simulink library "INT_EISGov_SelectParameter"  (R2016b)
settings: Solver=VariableStepAuto  StartTime=0.0  StopTime=10.0  RelTol=1e-3
settings Model: Creator=xuxingpei  LastModifiedBy=xuxingpei

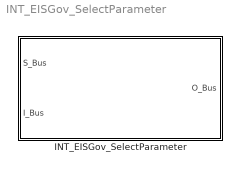
== system INT_EISGov_SelectParameter ==
  INT_EISGov_SelectParameter : Subsystem

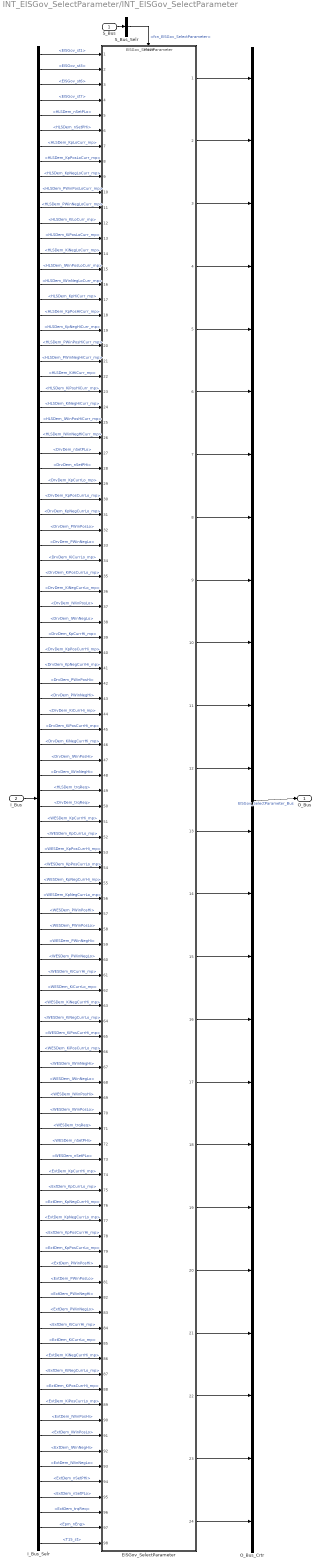
== system INT_EISGov_SelectParameter/INT_EISGov_SelectParameter ==
  S_Bus : Inport
  I_Bus : Inport  Port=2
  EISGov_SelectParameter : ModelReference  ModelNameDialog=EISGov_SelectParameter  SimulationMode=Normal  ModelReferenceVersion=1.180  TriggerPortName=function  TriggerPortTriggerType=function-call  TriggerPortStatesWhenEnabling=held
  I_Bus_Selr : BusSelector  OutputSignals=EISGov_st1,EISGov_st3,EISGov_st6,EISGov_st7,HLSDem_nSetPLo,HLSDem_nSetPHi,HLSDem_KpLoCurr_mp,HLSDem_KpPosLoCurr_mp,HLSDem_KpNegLoCurr_mp,HLSDem_PWinPosLoCurr_mp,HLSDem_PWinNegLoCurr_mp,HLSDem_KiLoCurr_mp,HLSDem_KiPosLoCurr_mp,HLSDem_KiNegLoCurr_mp,HLSDem_IWinPosLoCurr_mp,HLSDem_IWinNegLoCurr_mp,HLSDem_KpHiCurr_mp,HLSDem_KpPosHiCurr_mp,HLSDem_KpNegHiCurr_mp,HLSDem_PWinPosHiCurr_mp,HLSDem_PWinNegHiCurr_mp,HLSDem_KiHiCurr_mp,HLSDem_KiPosHiCurr_mp,HLSDem_KiNegHiCurr_mp,HLSDem_IWinPosHiCurr_mp,HLSDem_IWinNegHiCurr_mp,DrvDem_nSetPLo,DrvDem_nSetPHi,DrvDem_KpCurrLo_mp,DrvDem_KpPosCurrLo_mp,DrvDem_KpNegCurrLo_mp,DrvDem_PWinPosLo,DrvDem_PWinNegLo,DrvDem_KiCurrLo_mp,DrvDem_KiPosCurrLo_mp,DrvDem_KiNegCurrLo_mp,DrvDem_IWinPosLo,DrvDem_IWinNegLo,DrvDem_KpCurrHi_mp,DrvDem_KpPosCurrHi_mp,DrvDem_KpNegCurrHi_mp,DrvDem_PWinPosHi,DrvDem_PWinNegHi,DrvDem_KiCurrHi_mp,DrvDem_KiPosCurrHi_mp,DrvDem_KiNegCurrHi_mp,DrvDem_IWinPosHi,DrvDem_IWinNegHi,HLSDem_trqReq,DrvDem_trqReq,WESDem_KpCurrHi_mp,WESDem_KpCurrLo_mp,WESDem_KpPosCurrHi_mp,WESDem_KpPosCurrLo_mp,WESDem_KpNegCurrHi_mp,WESDem_KpNegCurrLo_mp,WESDem_PWinPosHi,WESDem_PWinPosLo,WESDem_PWinNegHi,WESDem_PWinNegLo,WESDem_KiCurrHi_mp,WESDem_KiCurrLo_mp,WESDem_KiNegCurrHi_mp,WESDem_KiNegCurrLo_mp,WESDem_KiPosCurrHi_mp,WESDem_KiPosCurrLo_mp,WESDem_IWinNegHi,WESDem_IWinNegLo,WESDem_IWinPosHi,WESDem_IWinPosLo,WESDem_trqReq,WESDem_nSetPHi,WESDem_nSetPLo,ExtDem_KpCurrHi_mp,ExtDem_KpCurrLo_mp,ExtDem_KpNegCurrHi_mp,ExtDem_KpNegCurrLo_mp,ExtDem_KpPosCurrHi_mp,ExtDem_KpPosCurrLo_mp,ExtDem_PWinPosHi,ExtDem_PWinPosLo,ExtDem_PWinNegHi,ExtDem_PWinNegLo,ExtDem_KiCurrHi_mp,ExtDem_KiCurrLo_mp,ExtDem_KiNegCurrHi_mp,ExtDem_KiNegCurrLo_mp,ExtDem_KiPosCurrHi_mp,ExtDem_KiPosCurrLo_mp,ExtDem_IWinPosHi,ExtDem_IWinPosLo,ExtDem_IWinNegHi,ExtDem_IWinNegLo,ExtDem_nSetPHi,ExtDem_nSetPLo,ExtDem_trqReq,Epm_nEng,T15_st
  O_Bus_Crtr : BusCreator  Inputs=24
  S_Bus_Selr : BusSelector  OutputSignals=fcn_EISGov_SelectParameter
  O_Bus : Outport
  wires:
  S_Bus_Selr/1 -> EISGov_SelectParameter/Trigger  "<fcn_EISGov_SelectParameter>"
  S_Bus/1 -> S_Bus_Selr/1
  I_Bus/1 -> I_Bus_Selr/1
  I_Bus_Selr/1 -> EISGov_SelectParameter/1  "<EISGov_st1>"
  I_Bus_Selr/2 -> EISGov_SelectParameter/2  "<EISGov_st3>"
  I_Bus_Selr/3 -> EISGov_SelectParameter/3  "<EISGov_st6>"
  I_Bus_Selr/4 -> EISGov_SelectParameter/4  "<EISGov_st7>"
  I_Bus_Selr/5 -> EISGov_SelectParameter/5  "<HLSDem_nSetPLo>"
  I_Bus_Selr/6 -> EISGov_SelectParameter/6  "<HLSDem_nSetPHi>"
  I_Bus_Selr/7 -> EISGov_SelectParameter/7  "<HLSDem_KpLoCurr_mp>"
  I_Bus_Selr/8 -> EISGov_SelectParameter/8  "<HLSDem_KpPosLoCurr_mp>"
  I_Bus_Selr/9 -> EISGov_SelectParameter/9  "<HLSDem_KpNegLoCurr_mp>"
  I_Bus_Selr/10 -> EISGov_SelectParameter/10  "<HLSDem_PWinPosLoCurr_mp>"
  I_Bus_Selr/11 -> EISGov_SelectParameter/11  "<HLSDem_PWinNegLoCurr_mp>"
  I_Bus_Selr/12 -> EISGov_SelectParameter/12  "<HLSDem_KiLoCurr_mp>"
  I_Bus_Selr/13 -> EISGov_SelectParameter/13  "<HLSDem_KiPosLoCurr_mp>"
  I_Bus_Selr/14 -> EISGov_SelectParameter/14  "<HLSDem_KiNegLoCurr_mp>"
  I_Bus_Selr/15 -> EISGov_SelectParameter/15  "<HLSDem_IWinPosLoCurr_mp>"
  I_Bus_Selr/16 -> EISGov_SelectParameter/16  "<HLSDem_IWinNegLoCurr_mp>"
  I_Bus_Selr/17 -> EISGov_SelectParameter/17  "<HLSDem_KpHiCurr_mp>"
  I_Bus_Selr/18 -> EISGov_SelectParameter/18  "<HLSDem_KpPosHiCurr_mp>"
  I_Bus_Selr/19 -> EISGov_SelectParameter/19  "<HLSDem_KpNegHiCurr_mp>"
  I_Bus_Selr/20 -> EISGov_SelectParameter/20  "<HLSDem_PWinPosHiCurr_mp>"
  I_Bus_Selr/21 -> EISGov_SelectParameter/21  "<HLSDem_PWinNegHiCurr_mp>"
  I_Bus_Selr/22 -> EISGov_SelectParameter/22  "<HLSDem_KiHiCurr_mp>"
  I_Bus_Selr/23 -> EISGov_SelectParameter/23  "<HLSDem_KiPosHiCurr_mp>"
  I_Bus_Selr/24 -> EISGov_SelectParameter/24  "<HLSDem_KiNegHiCurr_mp>"
  I_Bus_Selr/25 -> EISGov_SelectParameter/25  "<HLSDem_IWinPosHiCurr_mp>"
  I_Bus_Selr/26 -> EISGov_SelectParameter/26  "<HLSDem_IWinNegHiCurr_mp>"
  I_Bus_Selr/27 -> EISGov_SelectParameter/27  "<DrvDem_nSetPLo>"
  I_Bus_Selr/28 -> EISGov_SelectParameter/28  "<DrvDem_nSetPHi>"
  I_Bus_Selr/29 -> EISGov_SelectParameter/29  "<DrvDem_KpCurrLo_mp>"
  I_Bus_Selr/30 -> EISGov_SelectParameter/30  "<DrvDem_KpPosCurrLo_mp>"
  I_Bus_Selr/31 -> EISGov_SelectParameter/31  "<DrvDem_KpNegCurrLo_mp>"
  I_Bus_Selr/32 -> EISGov_SelectParameter/32  "<DrvDem_PWinPosLo>"
  I_Bus_Selr/33 -> EISGov_SelectParameter/33  "<DrvDem_PWinNegLo>"
  I_Bus_Selr/34 -> EISGov_SelectParameter/34  "<DrvDem_KiCurrLo_mp>"
  I_Bus_Selr/35 -> EISGov_SelectParameter/35  "<DrvDem_KiPosCurrLo_mp>"
  I_Bus_Selr/36 -> EISGov_SelectParameter/36  "<DrvDem_KiNegCurrLo_mp>"
  I_Bus_Selr/37 -> EISGov_SelectParameter/37  "<DrvDem_IWinPosLo>"
  I_Bus_Selr/38 -> EISGov_SelectParameter/38  "<DrvDem_IWinNegLo>"
  I_Bus_Selr/39 -> EISGov_SelectParameter/39  "<DrvDem_KpCurrHi_mp>"
  I_Bus_Selr/40 -> EISGov_SelectParameter/40  "<DrvDem_KpPosCurrHi_mp>"
  I_Bus_Selr/41 -> EISGov_SelectParameter/41  "<DrvDem_KpNegCurrHi_mp>"
  I_Bus_Selr/42 -> EISGov_SelectParameter/42  "<DrvDem_PWinPosHi>"
  I_Bus_Selr/43 -> EISGov_SelectParameter/43  "<DrvDem_PWinNegHi>"
  I_Bus_Selr/44 -> EISGov_SelectParameter/44  "<DrvDem_KiCurrHi_mp>"
  I_Bus_Selr/45 -> EISGov_SelectParameter/45  "<DrvDem_KiPosCurrHi_mp>"
  I_Bus_Selr/46 -> EISGov_SelectParameter/46  "<DrvDem_KiNegCurrHi_mp>"
  I_Bus_Selr/47 -> EISGov_SelectParameter/47  "<DrvDem_IWinPosHi>"
  I_Bus_Selr/48 -> EISGov_SelectParameter/48  "<DrvDem_IWinNegHi>"
  I_Bus_Selr/49 -> EISGov_SelectParameter/49  "<HLSDem_trqReq>"
  I_Bus_Selr/50 -> EISGov_SelectParameter/50  "<DrvDem_trqReq>"
  I_Bus_Selr/51 -> EISGov_SelectParameter/51  "<WESDem_KpCurrHi_mp>"
  I_Bus_Selr/52 -> EISGov_SelectParameter/52  "<WESDem_KpCurrLo_mp>"
  I_Bus_Selr/53 -> EISGov_SelectParameter/53  "<WESDem_KpPosCurrHi_mp>"
  I_Bus_Selr/54 -> EISGov_SelectParameter/54  "<WESDem_KpPosCurrLo_mp>"
  I_Bus_Selr/55 -> EISGov_SelectParameter/55  "<WESDem_KpNegCurrHi_mp>"
  I_Bus_Selr/56 -> EISGov_SelectParameter/56  "<WESDem_KpNegCurrLo_mp>"
  I_Bus_Selr/57 -> EISGov_SelectParameter/57  "<WESDem_PWinPosHi>"
  I_Bus_Selr/58 -> EISGov_SelectParameter/58  "<WESDem_PWinPosLo>"
  I_Bus_Selr/59 -> EISGov_SelectParameter/59  "<WESDem_PWinNegHi>"
  I_Bus_Selr/60 -> EISGov_SelectParameter/60  "<WESDem_PWinNegLo>"
  I_Bus_Selr/61 -> EISGov_SelectParameter/61  "<WESDem_KiCurrHi_mp>"
  I_Bus_Selr/62 -> EISGov_SelectParameter/62  "<WESDem_KiCurrLo_mp>"
  I_Bus_Selr/63 -> EISGov_SelectParameter/63  "<WESDem_KiNegCurrHi_mp>"
  I_Bus_Selr/64 -> EISGov_SelectParameter/64  "<WESDem_KiNegCurrLo_mp>"
  I_Bus_Selr/65 -> EISGov_SelectParameter/65  "<WESDem_KiPosCurrHi_mp>"
  I_Bus_Selr/66 -> EISGov_SelectParameter/66  "<WESDem_KiPosCurrLo_mp>"
  I_Bus_Selr/67 -> EISGov_SelectParameter/67  "<WESDem_IWinNegHi>"
  I_Bus_Selr/68 -> EISGov_SelectParameter/68  "<WESDem_IWinNegLo>"
  I_Bus_Selr/69 -> EISGov_SelectParameter/69  "<WESDem_IWinPosHi>"
  I_Bus_Selr/70 -> EISGov_SelectParameter/70  "<WESDem_IWinPosLo>"
  I_Bus_Selr/71 -> EISGov_SelectParameter/71  "<WESDem_trqReq>"
  I_Bus_Selr/72 -> EISGov_SelectParameter/72  "<WESDem_nSetPHi>"
  I_Bus_Selr/73 -> EISGov_SelectParameter/73  "<WESDem_nSetPLo>"
  I_Bus_Selr/74 -> EISGov_SelectParameter/74  "<ExtDem_KpCurrHi_mp>"
  I_Bus_Selr/75 -> EISGov_SelectParameter/75  "<ExtDem_KpCurrLo_mp>"
  I_Bus_Selr/76 -> EISGov_SelectParameter/76  "<ExtDem_KpNegCurrHi_mp>"
  I_Bus_Selr/77 -> EISGov_SelectParameter/77  "<ExtDem_KpNegCurrLo_mp>"
  I_Bus_Selr/78 -> EISGov_SelectParameter/78  "<ExtDem_KpPosCurrHi_mp>"
  I_Bus_Selr/79 -> EISGov_SelectParameter/79  "<ExtDem_KpPosCurrLo_mp>"
  I_Bus_Selr/80 -> EISGov_SelectParameter/80  "<ExtDem_PWinPosHi>"
  I_Bus_Selr/81 -> EISGov_SelectParameter/81  "<ExtDem_PWinPosLo>"
  I_Bus_Selr/82 -> EISGov_SelectParameter/82  "<ExtDem_PWinNegHi>"
  I_Bus_Selr/83 -> EISGov_SelectParameter/83  "<ExtDem_PWinNegLo>"
  I_Bus_Selr/84 -> EISGov_SelectParameter/84  "<ExtDem_KiCurrHi_mp>"
  I_Bus_Selr/85 -> EISGov_SelectParameter/85  "<ExtDem_KiCurrLo_mp>"
  I_Bus_Selr/86 -> EISGov_SelectParameter/86  "<ExtDem_KiNegCurrHi_mp>"
  I_Bus_Selr/87 -> EISGov_SelectParameter/87  "<ExtDem_KiNegCurrLo_mp>"
  I_Bus_Selr/88 -> EISGov_SelectParameter/88  "<ExtDem_KiPosCurrHi_mp>"
  I_Bus_Selr/89 -> EISGov_SelectParameter/89  "<ExtDem_KiPosCurrLo_mp>"
  I_Bus_Selr/90 -> EISGov_SelectParameter/90  "<ExtDem_IWinPosHi>"
  I_Bus_Selr/91 -> EISGov_SelectParameter/91  "<ExtDem_IWinPosLo>"
  I_Bus_Selr/92 -> EISGov_SelectParameter/92  "<ExtDem_IWinNegHi>"
  I_Bus_Selr/93 -> EISGov_SelectParameter/93  "<ExtDem_IWinNegLo>"
  I_Bus_Selr/94 -> EISGov_SelectParameter/94  "<ExtDem_nSetPHi>"
  I_Bus_Selr/95 -> EISGov_SelectParameter/95  "<ExtDem_nSetPLo>"
  I_Bus_Selr/96 -> EISGov_SelectParameter/96  "<ExtDem_trqReq>"
  I_Bus_Selr/97 -> EISGov_SelectParameter/97  "<Epm_nEng>"
  I_Bus_Selr/98 -> EISGov_SelectParameter/98  "<T15_st>"
  O_Bus_Crtr/1 -> O_Bus/1  "EISGov_SelectParameter_Bus"
  EISGov_SelectParameter/1 -> O_Bus_Crtr/1
  EISGov_SelectParameter/2 -> O_Bus_Crtr/2
  EISGov_SelectParameter/3 -> O_Bus_Crtr/3
  EISGov_SelectParameter/4 -> O_Bus_Crtr/4
  EISGov_SelectParameter/5 -> O_Bus_Crtr/5
  EISGov_SelectParameter/6 -> O_Bus_Crtr/6
  EISGov_SelectParameter/7 -> O_Bus_Crtr/7
  EISGov_SelectParameter/8 -> O_Bus_Crtr/8
  EISGov_SelectParameter/9 -> O_Bus_Crtr/9
  EISGov_SelectParameter/10 -> O_Bus_Crtr/10
  EISGov_SelectParameter/11 -> O_Bus_Crtr/11
  EISGov_SelectParameter/12 -> O_Bus_Crtr/12
  EISGov_SelectParameter/13 -> O_Bus_Crtr/13
  EISGov_SelectParameter/14 -> O_Bus_Crtr/14
  EISGov_SelectParameter/15 -> O_Bus_Crtr/15
  EISGov_SelectParameter/16 -> O_Bus_Crtr/16
  EISGov_SelectParameter/17 -> O_Bus_Crtr/17
  EISGov_SelectParameter/18 -> O_Bus_Crtr/18
  EISGov_SelectParameter/19 -> O_Bus_Crtr/19
  EISGov_SelectParameter/20 -> O_Bus_Crtr/20
  EISGov_SelectParameter/21 -> O_Bus_Crtr/21
  EISGov_SelectParameter/22 -> O_Bus_Crtr/22
  EISGov_SelectParameter/23 -> O_Bus_Crtr/23
  EISGov_SelectParameter/24 -> O_Bus_Crtr/24
